simulink model "affectofbrake"  (R2018a)
settings: Solver=ode23tb  StartTime=0.0  StopTime=10  RelTol=1e-3
values from neighbouring files (symbols this model uses):
  L = 12    [Run_mohinh1_2.m]
  M = 4200    [Run_mohinh1_2.m]
undefined symbols (not defined in the file or in its folder): C1, C2, Cl1, Cl2, hg, K1, K2, Kl1, Kl2, M1, m1, M2, m2, M3, q0, S, sigbuilder_block
settings Model: Creator=admin  LastModifiedBy=admin
settings SolverCC: AlgebraicLoopSolver=LineSearch

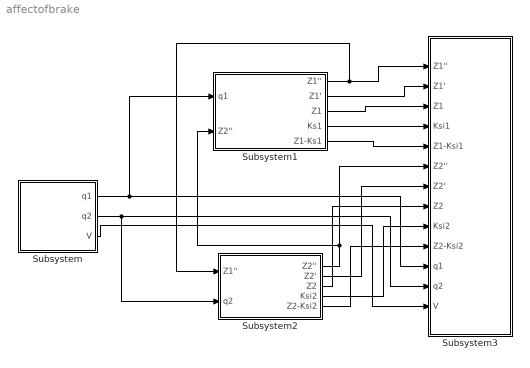
== system affectofbrake ==
  Subsystem : Subsystem
  Subsystem1 : Subsystem
  Subsystem2 : Subsystem
  Subsystem3 : Subsystem
  wires:
  Subsystem/1(q1) -> Subsystem1/1(q1), Subsystem3/11(q1)
  Subsystem/2(q2) -> Subsystem2/2(q2), Subsystem3/12(q2)
  Subsystem/3(V) -> Subsystem3/13(V)
  Subsystem2/1(Z2'') -> Subsystem3/6(Z2''), Subsystem1/2(Z2'')
  Subsystem1/1(Z1'') -> Subsystem2/1(Z1''), Subsystem3/1(Z1'')
  Subsystem1/2(Z1') -> Subsystem3/2(Z1')
  Subsystem1/3(Z1) -> Subsystem3/3(Z1)
  Subsystem1/4(Ks1) -> Subsystem3/4(Ksi1)
  Subsystem1/5(Z1-Ks1) -> Subsystem3/5(Z1-Ksi1)
  Subsystem2/2(Z2') -> Subsystem3/7(Z2')
  Subsystem2/3(Z2) -> Subsystem3/8(Z2)
  Subsystem2/4(Ksi2) -> Subsystem3/9(Ksi2)
  Subsystem2/5(Z2-Ksi2) -> Subsystem3/10(Z2-Ksi2)

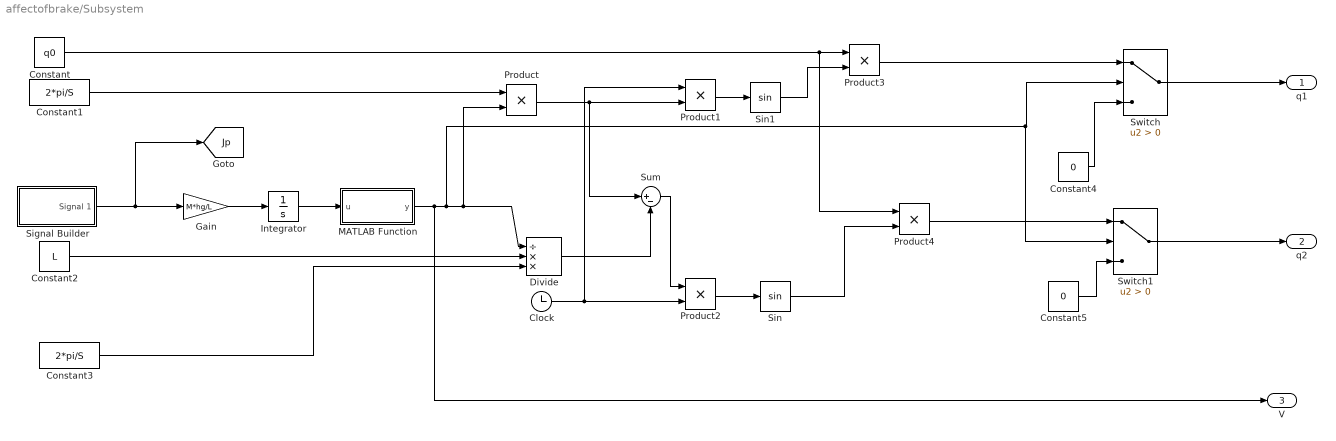
== system affectofbrake/Subsystem ==
  Clock : Clock
  Constant : Constant  Value=q0
  Constant1 : Constant  Value=2*pi/S
  Constant2 : Constant  Value=L
  Constant3 : Constant  Value=2*pi/S
  Constant4 : Constant  Value=0
  Constant5 : Constant  Value=0
  Divide : Product  Inputs=/**
  Gain : Gain  Gain=M*hg/L
  Integrator : Integrator
  MATLAB Function : MATLAB Function  TreatAsAtomicUnit=on
  Product{,1..4} (5 alike) : Product
  Signal Builder : Subsystem  Tag=STV Subsys  LoadFcn=sigbuilder_block('load');  StartFcn=sigbuilder_block('start');  StopFcn=sigbuilder_block('stop');  ClipboardFcn=sigbuilder_block('clipboard');  mask(Sigbuilder block){tuvar=[0:10]}
      mask help: Simulink:masks:SigbuilderBlock_MD
      mask init:
      | if ~strcmp(get_param(bdroot(gcbh),'SimulationStatus'),'stopped') tuvar = sigbuilder_block('maskInit'); end
      settings: CopyFcn=sigbuilder_block('copy');  DeleteFcn=sigbuilder_block('delete');  ModelCloseFcn=sigbuilder_block('modelClose');  PreSaveFcn=sigbuilder_block('preSave');  PauseFcn=sigbuilder_block('pause');  ContinueFcn=sigbuilder_block('continue');  NameChangeFcn=sigbuilder_block('namechange');  OpenFcn=sigbuilder_block('open',[437.6 199.2 550.4 400 ]);  CloseFcn=sigbuilder_block('close');
      mask Display: plot(0, 0, 100, 100,[2, 2, 32, 32, 2], [68, 8, 8, 68, 68],[32, 2], [38, 38], [32, 19, 2],[53, 60, 44], [32, 17, 17, 2],[16, 16, 31, 31]);txt = getActiveGroup(gcbh);text(2, 100, txt,'verticalAlignment', 'top');
  Sin : Trigonometry
  Sin1 : Trigonometry
  Sum : Sum  Inputs=|+-
  Switch : Switch  Criteria=u2 > Threshold
  Switch1 : Switch  Criteria=u2 > Threshold
  q1 : Outport
  q2 : Outport  Port=2
  V : Outport  Port=3
  tag scope: Jp=global
  wires:
  Signal Builder/1(Signal 1) -> [Jp], Gain/1
  Gain/1 -> Integrator/1
  Integrator/1 -> MATLAB Function/1(u)
  MATLAB Function/1(y) -> V/1, Switch1/2, Switch/2, Product/2, Divide/1
  Constant2/1 -> Divide/2
  Constant3/1 -> Divide/3
  Constant1/1 -> Product/1
  Product/1 -> Product1/2, Sum/1
  Sum/1 -> Product2/1
  Divide/1 -> Sum/2
  Clock/1 -> Product1/1, Product2/2
  Product2/1 -> Sin/1
  Product1/1 -> Sin1/1
  Sin1/1 -> Product3/2
  Constant/1 -> Product4/1, Product3/1
  Sin/1 -> Product4/2
  Product3/1 -> Switch/1
  Constant4/1 -> Switch/3
  Product4/1 -> Switch1/1
  Constant5/1 -> Switch1/3
  Switch/1 -> q1/1
  Switch1/1 -> q2/1

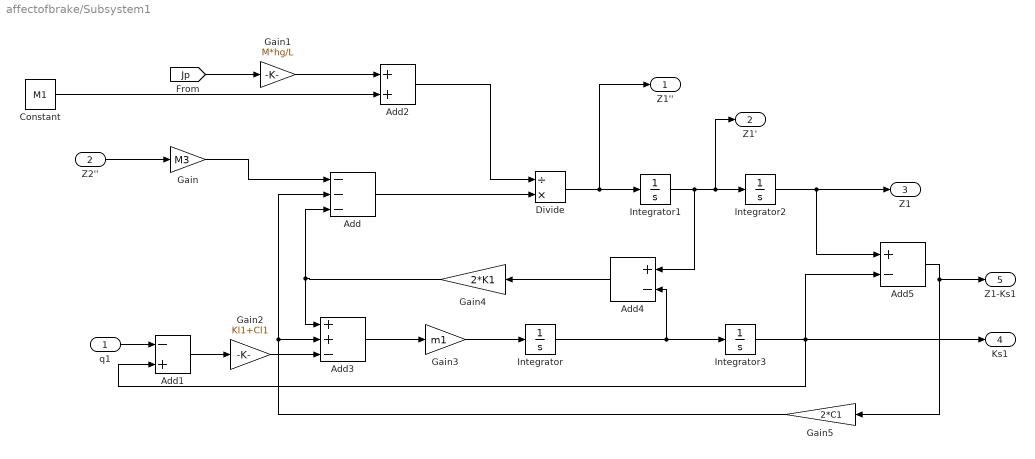
== system affectofbrake/Subsystem1 ==
  q1 : Inport
  Z2'' : Inport  Port=2
  Add : Sum  Inputs=---
  Add1 : Sum  Inputs=-+
  Add2 : Sum
  Add3 : Sum  Inputs=++-
  Add4 : Sum  Inputs=+-
  Add5 : Sum  Inputs=+-
  Constant : Constant  Value=M1
  Divide : Product  Inputs=/*
  Gain : Gain  Gain=M3
  Gain1 : Gain  Gain=M*hg/L
  Gain2 : Gain  Gain=Kl1+Cl1
  Gain3 : Gain  Gain=m1
  Gain4 : Gain  Gain=2*K1
  Gain5 : Gain  Gain=2*C1
  Integrator{,1..3} (4 alike) : Integrator
  Z1'' : Outport
  Z1' : Outport  Port=2
  Z1 : Outport  Port=3
  Ks1 : Outport  Port=4
  Z1-Ks1 : Outport  Port=5
  wires:
  Gain/1 -> Add/1
  q1/1 -> Add1/1
  [Jp] -> Gain1/1
  Gain1/1 -> Add2/1
  Constant/1 -> Add2/2
  Add1/1 -> Gain2/1
  Gain2/1 -> Add3/3
  Add3/1 -> Gain3/1
  Gain3/1 -> Integrator/1
  Add/1 -> Divide/2
  Add2/1 -> Divide/1
  Divide/1 -> Z1''/1, Integrator1/1
  Integrator1/1 -> Add4/1, Z1'/1, Integrator2/1
  Integrator2/1 -> Add5/1, Z1/1
  Add4/1 -> Gain4/1
  Integrator/1 -> Add4/2, Integrator3/1
  Integrator3/1 -> Add5/2, Add1/2, Ks1/1
  Add5/1 -> Z1-Ks1/1, Gain5/1
  Gain5/1 -> Add3/2, Add/2
  Gain4/1 -> Add3/1, Add/3
  Z2''/1 -> Gain/1

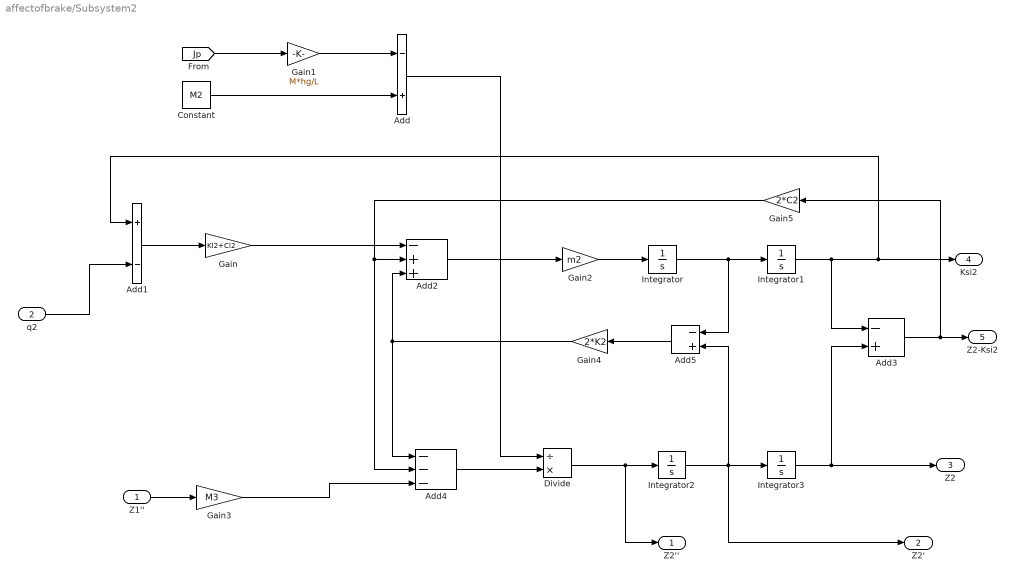
== system affectofbrake/Subsystem2 ==
  Z1'' : Inport
  q2 : Inport  Port=2
  Add : Sum  Inputs=-+
  Add1 : Sum  Inputs=+-
  Add2 : Sum  Inputs=-++
  Add3 : Sum  Inputs=-+
  Add4 : Sum  Inputs=---
  Add5 : Sum  Inputs=-+
  Constant : Constant  Value=M2
  Divide : Product  Inputs=/*
  Gain : Gain  Gain=Kl2+Cl2
  Gain1 : Gain  Gain=M*hg/L
  Gain2 : Gain  Gain=m2
  Gain3 : Gain  Gain=M3
  Gain4 : Gain  Gain=2*K2
  Gain5 : Gain  Gain=2*C2
  Integrator{,1..3} (4 alike) : Integrator
  Z2'' : Outport
  Z2' : Outport  Port=2
  Z2 : Outport  Port=3
  Ksi2 : Outport  Port=4
  Z2-Ksi2 : Outport  Port=5
  wires:
  [Jp] -> Gain1/1
  Gain1/1 -> Add/1
  Constant/1 -> Add/2
  Add1/1 -> Gain/1
  Gain/1 -> Add2/1
  Add2/1 -> Gain2/1
  Gain2/1 -> Integrator/1
  Integrator/1 -> Add5/1, Integrator1/1
  Integrator1/1 -> Add1/1, Ksi2/1, Add3/1
  q2/1 -> Add1/2
  Z1''/1 -> Gain3/1
  Gain3/1 -> Add4/3
  Add4/1 -> Divide/2
  Add/1 -> Divide/1
  Divide/1 -> Z2''/1, Integrator2/1
  Integrator2/1 -> Z2'/1, Add5/2, Integrator3/1
  Integrator3/1 -> Z2/1, Add3/2
  Add5/1 -> Gain4/1
  Gain4/1 -> Add2/3, Add4/1
  Add3/1 -> Gain5/1, Z2-Ksi2/1
  Gain5/1 -> Add4/2, Add2/2

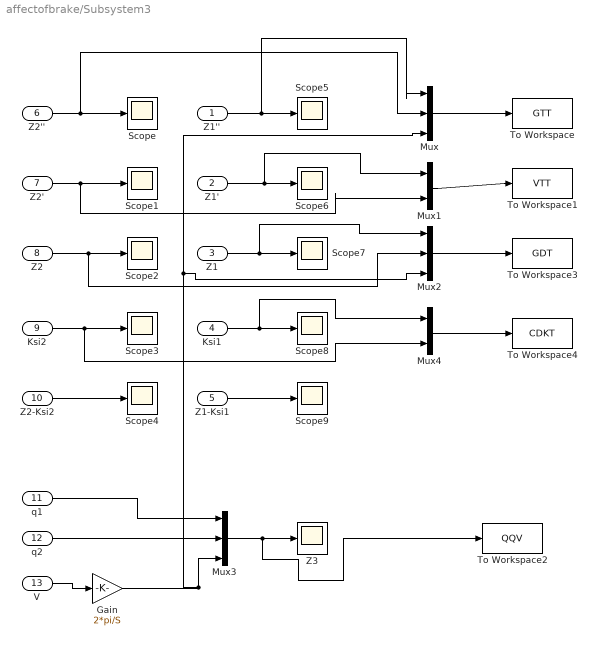
== system affectofbrake/Subsystem3 ==
  Z1'' : Inport
  Z1' : Inport  Port=2
  Z1 : Inport  Port=3
  Ksi1 : Inport  Port=4
  Z1-Ksi1 : Inport  Port=5
  Z2'' : Inport  Port=6
  Z2' : Inport  Port=7
  Z2 : Inport  Port=8
  Ksi2 : Inport  Port=9
  Z2-Ksi2 : Inport  Port=10
  q1 : Inport  Port=11
  q2 : Inport  Port=12
  V : Inport  Port=13
  Gain : Gain  Gain=2*pi/S
  Mux : Mux  Inputs=3
  Mux1 : Mux  Inputs=2
  Mux2 : Mux  Inputs=3
  Mux3 : Mux  Inputs=3
  Mux4 : Mux  Inputs=2
  Scope{,1..9} (10 alike) : Scope
  To Workspace : ToWorkspace  VariableName=GTT  SaveFormat=Timeseries  SampleTime=-1
  To Workspace1 : ToWorkspace  VariableName=VTT  SaveFormat=Timeseries  SampleTime=-1
  To Workspace2 : ToWorkspace  VariableName=QQV  SaveFormat=Timeseries  SampleTime=-1
  To Workspace3 : ToWorkspace  VariableName=GDT  SaveFormat=Timeseries  SampleTime=-1
  To Workspace4 : ToWorkspace  VariableName=CDKT  SaveFormat=Timeseries  SampleTime=-1
  Z3 : Scope
  wires:
  Mux/1 -> To Workspace/1
  Z1''/1 -> Mux/1, Scope5/1
  Z1'/1 -> Mux1/1, Scope6/1
  Mux1/1 -> To Workspace1/1
  Z1/1 -> Mux2/1, Scope7/1
  Ksi1/1 -> Mux4/1, Scope8/1
  Z1-Ksi1/1 -> Scope9/1
  Z2''/1 -> Mux/2, Scope/1
  Z2'/1 -> Mux1/2, Scope1/1
  Z2-Ksi2/1 -> Scope4/1
  q2/1 -> Mux3/2
  Gain/1 -> Mux3/3, Mux2/3, Mux/3
  q1/1 -> Mux3/1
  Mux3/1 -> To Workspace2/1, Z3/1
  Z2/1 -> Mux2/2, Scope2/1
  Ksi2/1 -> Mux4/2, Scope3/1
  Mux2/1 -> To Workspace3/1
  Mux4/1 -> To Workspace4/1
  V/1 -> Gain/1

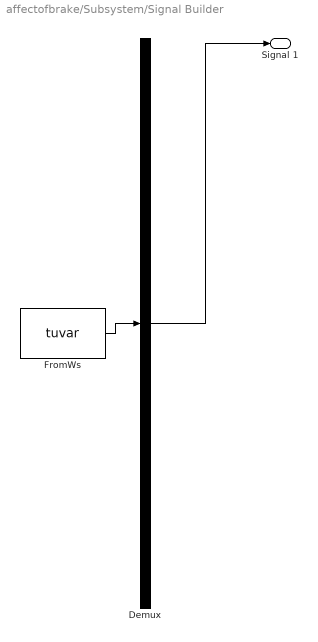
== system affectofbrake/Subsystem/Signal Builder ==
  Demux : Demux  Tag=STV Demux  Outputs=1
  FromWs : FromWorkspace  Tag=STV FromWs  VariableName=tuvar  SampleTime=0
      SigBuilderData=|
      | common.afterFinalStr = 'Extrapolate'
      | common.sampleTime = 0
      | dataSet.timeRange = [0 10]
      | dataSet.name = 'Group 1'
      | sbobj.Groups.Name = 'Group 1'
      | sbobj.Groups.Signals.Name = 'Signal 1'
      | sbobj.Groups.Signals.XData = [0 4 4 6 6 10]
      | sbobj.Groups.Signals.YData = [0 0 1 1 0 0]
  Signal 1 : Outport  Tag=STV Outport
  wires:
  Demux/1 -> Signal 1/1
  FromWs/1 -> Demux/1

== matlab function affectofbrake/Subsystem/MATLAB Function ==
  data: u input; y output
function y = fcn(u)

y = u;
